simulink model "automata_learning"  (R2022a)
settings: Solver=FixedStepAuto  StartTime=0.0  StopTime=10.0  FixedStep=0.01  RelTol=1e-3
settings Model: Creator=diego  LastModifiedBy=diego

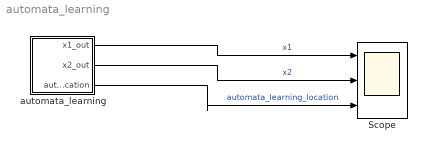
== system automata_learning ==
  Scope : Scope  NumInputPorts=3
  automata_learning : Stateflow chart  TreatAsAtomicUnit=on
  wires:
  automata_learning/1(x1_out) -> Scope/1  "x1"
  automata_learning/2(x2_out) -> Scope/2  "x2"
  automata_learning/3(automata_learning_location) -> Scope/3  "automata_learning_location"

== stateflow chart automata_learning/automata_learning ==
  settings: updateMethod=CONTINUOUS
  state loc1
    du:
    x1_dot = 0.0704534481999417 * x1 - 1.0682322679022036 * x2 - 0.15567711649509874;
    x2_dot = 0.8992468202686723 * x2 - 0.013011252348547941 * x1 + 1.9777609818411293;
    x1_out=x1;
    x2_out=x2;
    automata_learning_location =1;
  state loc2
    du:
    x1_dot = 0.04840411734767258 * x1 - 1.0018367484590271 * x2 + 0.0767735259660185;
    x2_dot = 6.452419820823707 * x1 - 0.019179947266934505 * x2 + 6.124703451030655;
    x1_out=x1;
    x2_out=x2;
    automata_learning_location =2;
  loc1 -> loc2 : [0.3288 * x1 - 0.333 * x2 + 1.0 < 0.0]
  (default) -> loc1 : {x1 = 1.0;
      | x2 = -1.0;}
  loc2 -> loc1 : [0.499 * x2 - 0.0006802 * x1 + 1.0 < 0.0]
  data: x1_out output; x1 local; x2_out output; x2 local; automata_learning_location output
  data x1 settings: updateMethod=SF_CONTINUOUS_TIME_DATA
  data x2 settings: updateMethod=SF_CONTINUOUS_TIME_DATA
